simulink model "cascade_realization"  (R2020b)
settings: Solver=VariableStepAuto  StartTime=0.0  StopTime=10.0  RelTol=1e-3
settings Model: Creator=user  LastModifiedBy=user

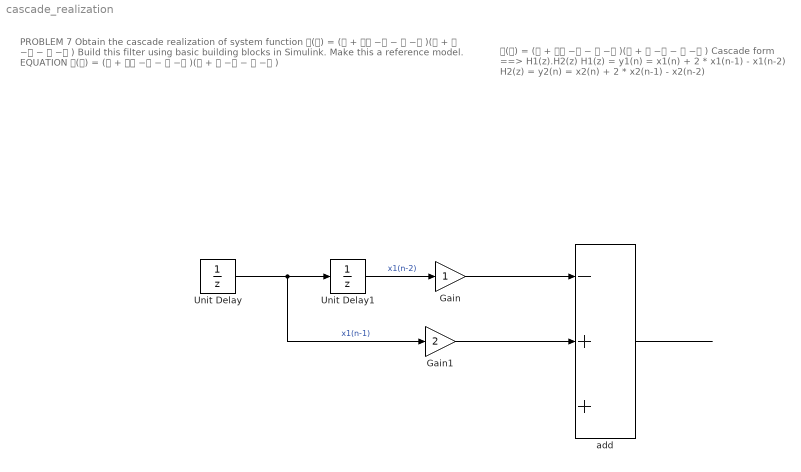
== system cascade_realization ==
  note: 𝐇(𝐳) = (𝟏 + 𝟐𝐳 −𝟏 − 𝐳 −𝟐 )(𝟏 + 𝐳 −𝟏 − 𝐳 −𝟐 )
      |
      | Cascade form ==> H1(z).H2(z)
      |
      | H1(z) = y1(n) = x1(n) + 2 * x1(n-1) - x1(n-2)
      | H2(z) = y2(n) = x2(n) + 2 * x2(n-1) - x2(n-2)
  note: PROBLEM 7
      |
      | Obtain the cascade realization of system function
      | 𝐇(𝐳) = (𝟏 + 𝟐𝐳 −𝟏 − 𝐳 −𝟐 )(𝟏 + 𝐳 −𝟏 − 𝐳 −𝟐 ) Build this filter using basic building blocks in Simulink. Make this a reference model.
      |
      | EQUATION
      | 𝐇(𝐳) = (𝟏 + 𝟐𝐳 −𝟏 − 𝐳 −𝟐 )(𝟏 + 𝐳 −𝟏 − 𝐳 −𝟐 )
  Gain : Gain
  Gain1 : Gain  Gain=2
  Unit Delay : UnitDelay  SampleTime=-1  HasFrameUpgradeWarning=on
  Unit Delay1 : UnitDelay  SampleTime=-1  HasFrameUpgradeWarning=on
  add : Sum  Inputs=-++
  wires:
  ? -> add/3, Unit Delay/1  "x1(n)"
  Unit Delay/1 -> Gain1/1, Unit Delay1/1  "x1(n-1)"
  Unit Delay1/1 -> Gain/1  "x1(n-2)"
  Gain/1 -> add/1
  Gain1/1 -> add/2
  add/1 -> ?
